simulink model "exciter_test"  (Simulink 6.0)
settings: Solver=ode3  StartTime=0.0  StopTime=10.0  FixedStep=0.01  RelTol=1e-3
settings Model: LastModifiedBy=Administrator

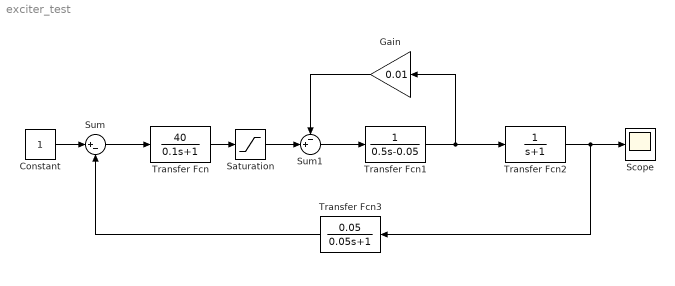
== system exciter_test ==
  Constant : Constant
  Gain : Gain  Orientation=left  Gain=0.01
  Saturation : Saturate  UpperLimit=30  LowerLimit=-30
  Scope : Scope
      settings: SaveName=y  DataFormat=Array
  Sum : Sum  Inputs=|+-
  Sum1 : Sum  Inputs=-+|
  Transfer Fcn : TransferFcn  Numerator=[40]  Denominator=[0.1 1]
  Transfer Fcn1 : TransferFcn  Denominator=[0.5 -0.05]
  Transfer Fcn2 : TransferFcn  Denominator=[1 1]
  Transfer Fcn3 : TransferFcn  Orientation=left  Numerator=[0.05]  Denominator=[0.05 1]
  wires:
  Constant/1 -> Sum/1
  Sum/1 -> Transfer Fcn/1
  Transfer Fcn/1 -> Saturation/1
  Sum1/1 -> Transfer Fcn1/1
  Transfer Fcn1/1 -> Transfer Fcn2/1, Gain/1
  Transfer Fcn3/1 -> Sum/2
  Saturation/1 -> Sum1/2
  Gain/1 -> Sum1/1
  Transfer Fcn2/1 -> Scope/1, Transfer Fcn3/1
